simulink model "practice_final_part_4"  (Simulink 8.3)
settings: Solver=ode45  StartTime=0.0  StopTime=20  RelTol=1e-3
undefined symbols (not defined in the file or in its folder): drawRodMass, P
settings Model: Creator=beard  LastModifiedBy=jhl48
settings DataIOCC: LimitDataPoints=off
settings OptimizationCC: ExpressionDepthLimit=2147483647
settings DebuggingCC: SolverPrmCheckMsg=none  FcnCallInpInsideContextMsg=UseLocalSettings

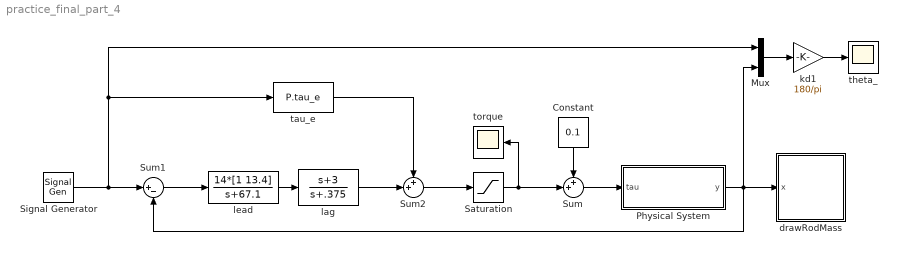
== system practice_final_part_4 ==
  Constant : Constant  Value=0.1
  Mux : Mux  Inputs=2
  Physical System : Subsystem
  Saturation : Saturate  UpperLimit=P.tau_max  LowerLimit=-P.tau_max
  Signal Generator : SignalGenerator  WaveForm=square  Amplitude=10*pi/180  Frequency=.1
  Sum : Sum  Inputs=++|
  Sum1 : Sum  Inputs=|+-
  Sum2 : Sum  Inputs=++|
  drawRodMass : Subsystem
      mask init:
      | % drawing parameters
      | L = 1;
      | w = 0.01;
      | R = 0.1;
      | H = 1;
      mask Display: image(imread('tv.jpg'))
  kd1 : Gain  Gain=180/pi
  lag : TransferFcn  Numerator=[1 3]  Denominator=[1 .375]
  lead : TransferFcn  Numerator=14*[1 13.4]  Denominator=[1 67.1]
  tau_e : Fcn  Expr=P.tau_e
  theta_ : Scope
      settings: YMin=-35  YMax=30
  torque : Scope
      settings: YMin=-0.65  YMax=0.2  SaveName=ScopeData2
  wires:
  Mux/1 -> kd1/1
  kd1/1 -> theta_/1
  Signal Generator/1 -> Sum1/1, tau_e/1, Mux/1
  Physical System/1(y) -> Sum1/2, drawRodMass/1(x), Mux/2
  Saturation/1 -> torque/1, Sum/2
  Sum/1 -> Physical System/1(tau)
  Constant/1 -> Sum/1
  lead/1 -> lag/1
  Sum1/1 -> lead/1
  lag/1 -> Sum2/2
  Sum2/1 -> Saturation/1
  tau_e/1 -> Sum2/1

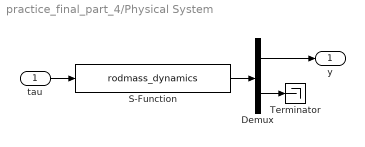
== system practice_final_part_4/Physical System ==
  tau : Inport
  Demux : Demux  Outputs=[1;2]
  S-Function : S-Function  FunctionName=rodmass_dynamics  Parameters=P  EnableBusSupport=off
  Terminator : Terminator
  y : Outport
  wires:
  tau/1 -> S-Function/1
  S-Function/1 -> Demux/1
  Demux/2 -> Terminator/1
  Demux/1 -> y/1

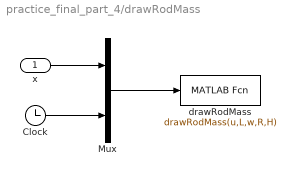
== system practice_final_part_4/drawRodMass ==
  x : Inport
  Clock : Clock
  Mux : Mux  Inputs=2
  drawRodMass : MATLABFcn  MATLABFcn=drawRodMass(u,L,w,R,H)  OutputDimensions=0  SampleTime=0.1
  wires:
  Clock/1 -> Mux/2
  x/1 -> Mux/1
  Mux/1 -> drawRodMass/1
